simulink model "ROLL_usporedba"  (R2020b)
settings: Solver=VariableStepAuto  StartTime=0.0  StopTime=10.0  RelTol=1e-3
undefined symbols (not defined in the file): k_r2, wn_r2, zeta_r2
settings Model: Creator=Ivan  LastModifiedBy=Ivan

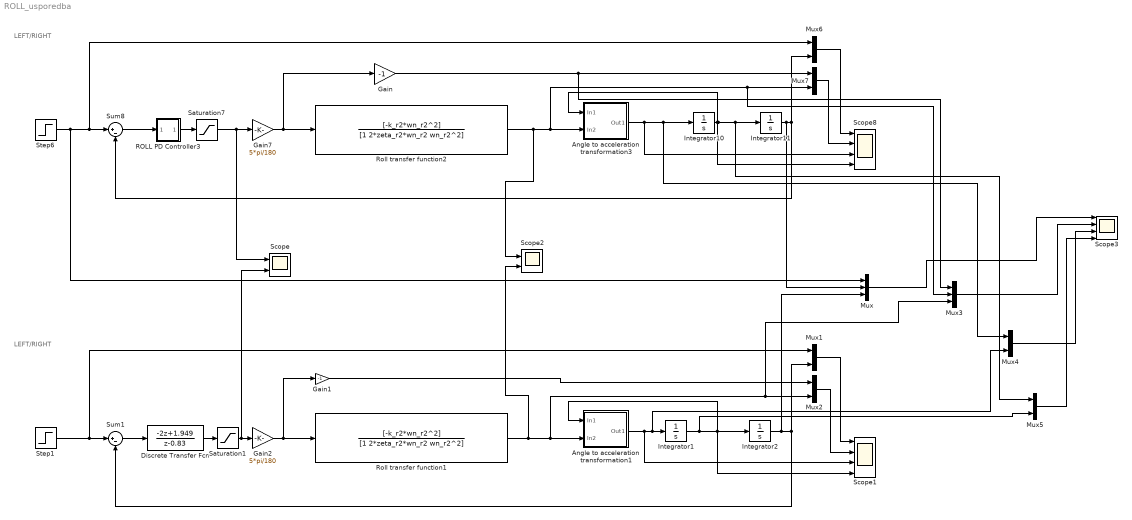
== system ROLL_usporedba ==
  note: LEFT/RIGHT
  note: LEFT/RIGHT
  Angle to acceleration transformation1 : Subsystem
  Angle to acceleration transformation3 : Subsystem
  Discrete Transfer Fcn : DiscreteTransferFcn  Numerator=[-2 1.949]  Denominator=[1 -0.83]  SampleTime=0.1
  Gain : Gain  Gain=-1
  Gain1 : Gain  Gain=-1
  Gain2 : Gain  Gain=5*pi/180
  Gain7 : Gain  Gain=5*pi/180
  Integrator{1..2,10..11} (4 alike) : Integrator
  Mux : Mux  Inputs=3
  Mux{1..2,4..7} (6 alike) : Mux  Inputs=2
  Mux3 : Mux  Inputs=3
  ROLL PD Controller3 : Subsystem
  Roll transfer function1 : TransferFcn  Numerator=[-k_r2*wn_r2^2]  Denominator=[1 2*zeta_r2*wn_r2 wn_r2^2]
  Roll transfer function2 : TransferFcn  Numerator=[-k_r2*wn_r2^2]  Denominator=[1 2*zeta_r2*wn_r2 wn_r2^2]
  Saturation1 : Saturate  UpperLimit=1  LowerLimit=-1
  Saturation7 : Saturate  UpperLimit=1  LowerLimit=-1
  Scope : Scope  NumInputPorts=2
  Scope1 : Scope  NumInputPorts=4
  Scope2 : Scope  NumInputPorts=2
  Scope3 : Scope  NumInputPorts=4
  Scope8 : Scope  NumInputPorts=4
  Step1 : Step  Time=0  After=2  SampleTime=0
  Step6 : Step  Time=0  After=2  SampleTime=0
  Sum1 : Sum  Inputs=|+-
  Sum8 : Sum  Inputs=|+-
  wires:
  Gain/1 -> Mux3/1, Mux7/1
  Mux7/1 -> Scope8/2
  Roll transfer function2/1 -> Scope2/1, Mux3/2, Mux7/2, Angle to acceleration transformation3/2(In2)
  Saturation7/1 -> Scope/1, Gain7/1
  ROLL PD Controller3/1(" ") -> Saturation7/1
  Mux6/1 -> Scope8/1
  Step6/1 -> Mux/1, Mux6/1, Sum8/1
  Sum8/1 -> ROLL PD Controller3/1("  ")
  Integrator10/1 -> Angle to acceleration transformation3/1(In1), Scope8/4, Mux5/1, Integrator11/1
  Integrator11/1 -> Mux/2, Mux6/2, Sum8/2
  Gain7/1 -> Gain/1, Roll transfer function2/1
  Angle to acceleration transformation3/1(Out1) -> Scope8/3, Mux4/1, Integrator10/1
  Gain1/1 -> Mux2/1
  Discrete Transfer Fcn/1 -> Saturation1/1
  Mux1/1 -> Scope1/1
  Gain2/1 -> Gain1/1, Roll transfer function1/1
  Saturation1/1 -> Scope/2, Gain2/1
  Mux2/1 -> Scope1/2
  Sum1/1 -> Discrete Transfer Fcn/1
  Roll transfer function1/1 -> Scope2/2, Mux3/3, Mux2/2, Angle to acceleration transformation1/2(In2)
  Angle to acceleration transformation1/1(Out1) -> Scope1/3, Mux4/2, Integrator1/1
  Integrator1/1 -> Mux5/2, Angle to acceleration transformation1/1(In1), Scope1/4, Integrator2/1
  Step1/1 -> Mux1/1, Sum1/1
  Integrator2/1 -> Mux/3, Mux1/2, Sum1/2
  Mux/1 -> Scope3/1
  Mux3/1 -> Scope3/2
  Mux4/1 -> Scope3/3
  Mux5/1 -> Scope3/4

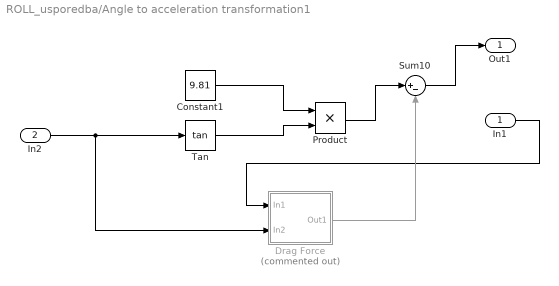
== system ROLL_usporedba/Angle to acceleration transformation1 ==
  In1 : Inport
  In2 : Inport  Port=2
  Constant1 : Constant  Value=9.81
  Drag Force : Subsystem  Commented=on
  Product : Product
  Sum10 : Sum  Inputs=|+-
  Tan : Trigonometry  Operator=tan
  Out1 : Outport
  wires:
  In2/1 -> Drag Force/2(In2), Tan/1
  Constant1/1 -> Product/1
  Tan/1 -> Product/2
  Product/1 -> Sum10/1
  Sum10/1 -> Out1/1
  In1/1 -> Drag Force/1(In1)
  Drag Force/1(Out1) -> Sum10/2

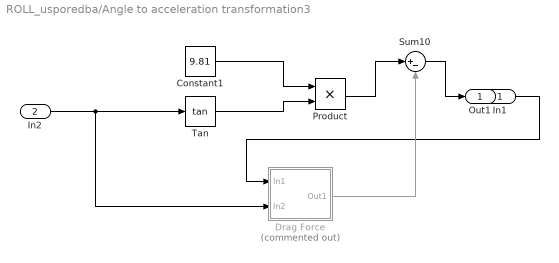
== system ROLL_usporedba/Angle to acceleration transformation3 ==
  In1 : Inport
  In2 : Inport  Port=2
  Constant1 : Constant  Value=9.81
  Drag Force : Subsystem  Commented=on
  Product : Product
  Sum10 : Sum  Inputs=|+-
  Tan : Trigonometry  Operator=tan
  Out1 : Outport
  wires:
  In2/1 -> Drag Force/2(In2), Tan/1
  Constant1/1 -> Product/1
  Tan/1 -> Product/2
  Product/1 -> Sum10/1
  Sum10/1 -> Out1/1
  In1/1 -> Drag Force/1(In1)
  Drag Force/1(Out1) -> Sum10/2

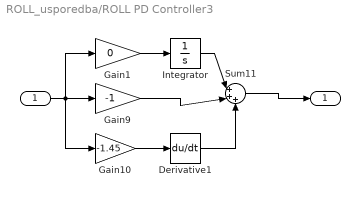
== system ROLL_usporedba/ROLL PD Controller3 ==
  "  " : Inport
  Derivative1 : Derivative
  Gain1 : Gain  Gain=0
  Gain10 : Gain  Gain=-1.45
  Gain9 : Gain  Gain=-1
  Integrator : Integrator
  Sum11 : Sum  Inputs=|+++
  " " : Outport
  wires:
  Gain9/1 -> Sum11/2
  Gain10/1 -> Derivative1/1
  "  "/1 -> Gain1/1, Gain10/1, Gain9/1
  Derivative1/1 -> Sum11/3
  Sum11/1 -> " "/1
  Integrator/1 -> Sum11/1
  Gain1/1 -> Integrator/1

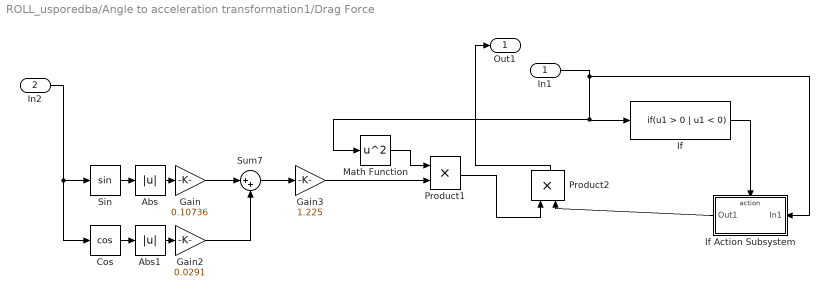
== system ROLL_usporedba/Angle to acceleration transformation1/Drag Force ==
  In1 : Inport
  In2 : Inport  Port=2
  Abs : Abs
  Abs1 : Abs
  Cos : Trigonometry  Operator=cos
  Gain : Gain  Gain=0.10736
  Gain2 : Gain  Gain=0.0291
  Gain3 : Gain  Gain=1.225
  If : If  IfExpression=u1 > 0 | u1 < 0  ShowElse=off
  If Action Subsystem : Subsystem  TreatAsAtomicUnit=on
  Math Function : Math  Operator=square  SaturateOnIntegerOverflow=on
  Product1 : Product
  Product2 : Product
  Sin : Trigonometry
  Sum7 : Sum  Inputs=|++
  Out1 : Outport
  wires:
  In1/1 -> If Action Subsystem/1(In1), Math Function/1, If/1
  Cos/1 -> Abs1/1
  Gain3/1 -> Product1/2
  Product2/1 -> Out1/1
  Sum7/1 -> Gain3/1
  In2/1 -> Sin/1, Cos/1
  Abs1/1 -> Gain2/1
  Gain2/1 -> Sum7/2
  Math Function/1 -> Product1/1
  Sin/1 -> Abs/1
  Product1/1 -> Product2/1
  Gain/1 -> Sum7/1
  Abs/1 -> Gain/1
  If/1 -> If Action Subsystem/Action
  If Action Subsystem/1(Out1) -> Product2/2

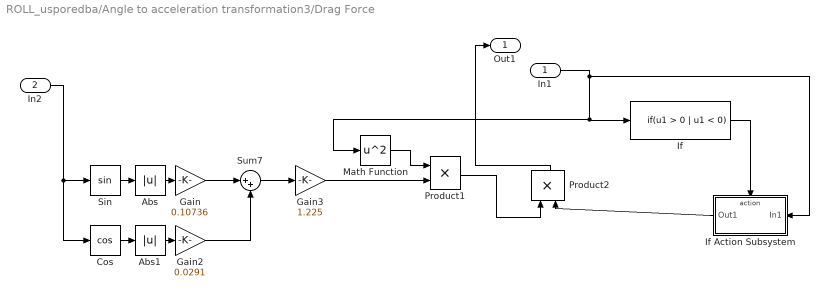
== system ROLL_usporedba/Angle to acceleration transformation3/Drag Force ==
  In1 : Inport
  In2 : Inport  Port=2
  Abs : Abs
  Abs1 : Abs
  Cos : Trigonometry  Operator=cos
  Gain : Gain  Gain=0.10736
  Gain2 : Gain  Gain=0.0291
  Gain3 : Gain  Gain=1.225
  If : If  IfExpression=u1 > 0 | u1 < 0  ShowElse=off
  If Action Subsystem : Subsystem  TreatAsAtomicUnit=on
  Math Function : Math  Operator=square  SaturateOnIntegerOverflow=on
  Product1 : Product
  Product2 : Product
  Sin : Trigonometry
  Sum7 : Sum  Inputs=|++
  Out1 : Outport
  wires:
  In1/1 -> If Action Subsystem/1(In1), Math Function/1, If/1
  Cos/1 -> Abs1/1
  Gain3/1 -> Product1/2
  Product2/1 -> Out1/1
  Sum7/1 -> Gain3/1
  In2/1 -> Sin/1, Cos/1
  Abs1/1 -> Gain2/1
  Gain2/1 -> Sum7/2
  Math Function/1 -> Product1/1
  Sin/1 -> Abs/1
  Product1/1 -> Product2/1
  Gain/1 -> Sum7/1
  Abs/1 -> Gain/1
  If/1 -> If Action Subsystem/Action
  If Action Subsystem/1(Out1) -> Product2/2

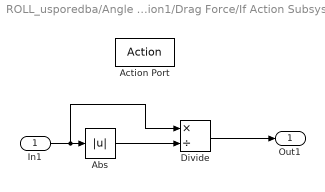
== system ROLL_usporedba/Angle to acceleration transformation1/Drag Force/If Action Subsystem ==
  In1 : Inport
  Action Port : ActionPort
  Abs : Abs
  Divide : Product  Inputs=*/
  Out1 : Outport
  wires:
  Abs/1 -> Divide/2
  In1/1 -> Divide/1, Abs/1
  Divide/1 -> Out1/1

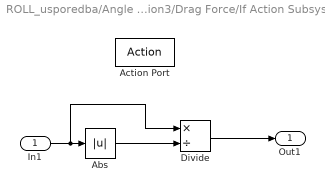
== system ROLL_usporedba/Angle to acceleration transformation3/Drag Force/If Action Subsystem ==
  In1 : Inport
  Action Port : ActionPort
  Abs : Abs
  Divide : Product  Inputs=*/
  Out1 : Outport
  wires:
  Abs/1 -> Divide/2
  In1/1 -> Divide/1, Abs/1
  Divide/1 -> Out1/1
